simulink model "GVCU_HIL_simscape"  (R2026a)
settings: Solver=ode3  StartTime=0  StopTime=10  FixedStep=0.001
model workspace (MAT data in the model file):
  CANoelibParameters : object (value not decoded)
values from neighbouring files (symbols this model uses):
  acc_pedal_data = pedal_data.accelerator_pedal_position_t0    [Init_Simscape_main.m]
  acc_pedal_time = pedal_data.t0    [Init_Simscape_main.m]
  brk_pedal_data = brake_pedal_data.shared_brakes_drvrBrkPedlPerc_t0    [Init_Simscape_main.m]
  brk_pedal_time = brake_pedal_data.t0    [Init_Simscape_main.m]
  cycle_len = zeros(1, num_cycles)    [Init_Simscape_main.m]
  cycle_speed_matrix = zeros(max_cycle_len, num_cycles)    [Init_Simscape_main.m]
  cycle_time_matrix = zeros(max_cycle_len, num_cycles)    [Init_Simscape_main.m]
  veh_speed_data = speed_data.shared_dynamicsVso_vehVelLgt_t0    [Init_Simscape_main.m]
  veh_speed_time = speed_data.t0    [Init_Simscape_main.m]
undefined symbols (not defined in the file or in its folder): Active, aero, AuxActive, bat, brake, config, environment, FL, FL_prs_voltage, FR, FR_prs_voltage, front, pos, powertrain, rear, RL, RL_prs_voltage, RR, RR_prs_voltage, tir, veh, VGetRawValueFlag, Voltage, VT2816_1_Ch1, VT2816_1_Ch2, VT2816_1_Ch3, VT2816_1_Ch4, VT2816_3_Ch13, VT2816_3_Ch14, VT7101_1_Out2, VTS, X, Y, Z
libraries: sm_lib x358, fl_lib x272, nesl_utility x193, canoelib x127, sdl_lib x36, autolibsharedcoupling x21, autolibcoupling x9, slpidlib x7, simulink x3, autolibshareddiff x3, autolibshared x3, autolibutils x1
(part 10 of 17)

== system GVCU_HIL_simscape/GVCU - HiL/Commented messages/Message Output9 ==
  In1 : Inport
  Bus Selector : BusSelector  OutputSignals=charge_current,charge_port_status,charge_voltage,charging_mode,e2e_alive_counter_disabled,e2e_checksum_disabled,evcc_status,inlet_motor_status,obc_fan_req,obc_pump_req,obc_status
  S-Function_1 : S-Function  FunctionName=sigout  Parameters=dbName;nodeName;msgName;11;'charge_current';'charge_port_status';'charge_voltage';'charging_mode';'e2e_alive_counter_disabled';'e2e_checksum_disabled';'evcc_status';'inlet_motor_status';'obc_fan_req';'obc_pump_req';'obc_status';VGetRawValueFlag(rawValue);'inherited'  SFunctionDeploymentMode=off  EnableBusSupport=off
      settings: AttributesFormatString=charge_current\ncharge_port_status\ncharge_voltage\ncharging_mode\ne2e_alive_counter_disabled\ne2e_checksum_disabled\nevcc_status\ninlet_motor_status\nobc_fan_req\nobc_pump_req\nobc_status\n
  wires:
  In1/1 -> Bus Selector/1
  Bus Selector/1 -> S-Function_1/1  "<charge_current>"
  Bus Selector/2 -> S-Function_1/2  "<charge_port_status>"
  Bus Selector/3 -> S-Function_1/3  "<charge_voltage>"
  Bus Selector/4 -> S-Function_1/4  "<charging_mode>"
  Bus Selector/5 -> S-Function_1/5  "<e2e_alive_counter_disabled>"
  Bus Selector/6 -> S-Function_1/6  "<e2e_checksum_disabled>"
  Bus Selector/7 -> S-Function_1/7  "<evcc_status>"
  Bus Selector/8 -> S-Function_1/8  "<inlet_motor_status>"
  Bus Selector/9 -> S-Function_1/9  "<obc_fan_req>"
  Bus Selector/10 -> S-Function_1/10  "<obc_pump_req>"
  Bus Selector/11 -> S-Function_1/11  "<obc_status>"

== system GVCU_HIL_simscape/Powertrain (EV)/AWD_Powertrain1/Central axle ==
  Rear_axle_speed : Inport
  Tosional_rear_c : Inport  Port=2
  Central_Clutch : autolibcoupling/Disc Clutch  port_config=Simulink  Reff=.091/2  Ndisk=9  Aeff=0.006283185  Peng=320000  Jin=.1  Jout=.1  muk=.088  mus=.089  bin=.001  bout=.001  win_o=pos.xdot_0/veh.TyreLoadedRadius_F*veh.BevelGear_F  wout_o=pos.xdot_0/veh.TyreLoadedRadius_F*veh.BevelGear_F  tauC=.01  InitiallyLocked=off  maxAbsSpd=3000  blkID=1
  FR1 : autolibsharedcoupling/Torsional Compliance  port_config=Simulink  extInfo=off  k=5e4  b=4e2  theta_o=0  domega_o=0  omega_c=3000  blkID=0  aMode=1
  FR2 : autolibsharedcoupling/Torsional Compliance  port_config=Simulink  extInfo=off  k=5e4  b=4e2  theta_o=0  domega_o=0  omega_c=3000  blkID=0  aMode=1
  Gain1 : Gain  Gain=1/0.93
  Terminator : Terminator
  drop gear + omega_to_rpm_central : Gain  Gain=0.92 *30/pi
  Prop_shaft_trq : Outport
  Central_axle_trq : Outport  Port=2
  tag scope: third_shaft_spd=global
  wires:
  Central_Clutch/1 -> Terminator/1
  [Center_prs] -> Central_Clutch/1
  FR2/2 -> Central_Clutch/2
  Gain1/1 -> Prop_shaft_trq/1
  FR1/2 -> Gain1/1
  Tosional_rear_c/1 -> drop gear + omega_to_rpm_central/1, FR1/2
  FR2/1 -> Central_axle_trq/1
  FR1/1 -> Central_Clutch/3
  Central_Clutch/3 -> FR1/1
  Central_Clutch/2 -> FR2/2  "FrontSpd"
  Rear_axle_speed/1 -> FR2/1
  drop gear + omega_to_rpm_central/1 -> [third_shaft_spd]  "Front_axle_freq"

== system GVCU_HIL_simscape/Powertrain (EV)/AWD_Powertrain1/Front Axle ==
  AxlSpd : Inport
  Veh : Inport  Port=2
  Bus Selector : BusSelector  OutputSignals=Wheels.Omega
  Demux : Demux
  FL : autolibsharedcoupling/Torsional Compliance  port_config=Simulink  extInfo=off  k=5e4  b=4e2  theta_o=0  domega_o=0  omega_c=3000  blkID=0  aMode=1
  FL_Clutch : autolibcoupling/Disc Clutch  port_config=Simulink  Reff=.091/2  Ndisk=9  Aeff=0.006283185  Peng=320000  Jin=.1  Jout=.1  muk=.088  mus=.089  bin=.001  bout=.001  win_o=pos.xdot_0/veh.TyreLoadedRadius_F  wout_o=pos.xdot_0/veh.TyreLoadedRadius_F  tauC=1  InitiallyLocked=off  maxAbsSpd=3000  blkID=1
  FR : autolibsharedcoupling/Torsional Compliance  port_config=Simulink  extInfo=off  k=5e4  b=4e2  theta_o=0  domega_o=0  omega_c=3000  blkID=0  aMode=1
  FR_Clutch : autolibcoupling/Disc Clutch  port_config=Simulink  Reff=.091/2  Ndisk=9  Aeff=0.006283185  Peng=320000  Jin=.1  Jout=.1  muk=.088  mus=.089  bin=.001  bout=.001  win_o=pos.xdot_0/veh.TyreLoadedRadius_F  wout_o=pos.xdot_0/veh.TyreLoadedRadius_F  tauC=.01  InitiallyLocked=off  maxAbsSpd=3000  blkID=1
  Gain : Gain  Gain=1/2.71
  Split Torsional Compliance : autolibsharedcoupling/Split Torsional Compliance  port_config=Simulink  cplrMode=Shaft split  extInfo=off  k1=5e4  b1=4e2  omega1_c=1000  theta1_o=0  domega1_o=0  k2=5e4  b2=4e2  omega2_c=1000  theta2_o=0  domega2_o=0  blkID=0  aMode=1
      settings: LibrarySourceBlock=autolibcoupling/Split Torsional Compliance
  Terminator{,1..3} (4 alike) : Terminator
  omega_to_freq_FL : Gain  Gain=98/(2*pi)
  omega_to_freq_FR : Gain  Gain=98/(2*pi)
  Split torsional Compliance Trq : Outport
  Trq_FL : Outport  Port=2
  Trq_FR : Outport  Port=3
  tag scope: Axl_front_Spd=global, FL_G_Spd=global, FL_R_Spd=global, FL_sen=global, FR_G_Spd=global, FR_R_Spd=global, FR_sen=global, Split_tors_FL=global, Split_tors_FR=global
  wires:
  Split Torsional Compliance/1 -> Split torsional Compliance Trq/1
  FR/2 -> Trq_FR/1
  FL/2 -> Trq_FL/1
  FR/1 -> FR_Clutch/3
  FL/1 -> FL_Clutch/3
  FL_Clutch/1 -> Terminator3/1
  FR_Clutch/1 -> Terminator2/1
  FR_Clutch/2 -> Split Torsional Compliance/3
  FL_Clutch/2 -> Split Torsional Compliance/2
  Demux/2 -> [FR_G_Spd], FR/2
  FR_Clutch/3 -> omega_to_freq_FR/1, [FR_R_Spd], FR/1
  Demux/4 -> Terminator1/1
  Demux/3 -> Terminator/1
  Bus Selector/1 -> Demux/1  "<Omega>"
  Veh/1 -> Bus Selector/1
  FL_Clutch/3 -> omega_to_freq_FL/1, [FL_R_Spd], FL/1
  [FR_prs] -> FR_Clutch/1
  [FL_prs] -> FL_Clutch/1
  Split Torsional Compliance/2 -> [Split_tors_FL], FL_Clutch/2  "Front_left_clutch"
  AxlSpd/1 -> Gain/1
  Split Torsional Compliance/3 -> [Split_tors_FR], FR_Clutch/2  "Front_right_clutch"
  omega_to_freq_FL/1 -> [FL_sen]  "FL_freq"
  omega_to_freq_FR/1 -> [FR_sen]  "FR_freq"
  Demux/1 -> [FL_G_Spd], FL/2
  Gain/1 -> [Axl_front_Spd], Split Torsional Compliance/1  "Front axle"

== system GVCU_HIL_simscape/Powertrain (EV)/AWD_Powertrain1/Rear Axle ==
  Prop_shaft_trq : Inport
  Veh : Inport  Port=2
  Bus Selector : BusSelector  OutputSignals=Wheels.Omega
  Demux : Demux
  Gain{,1..3} (4 alike) : Gain  Gain=37/(2*pi)
  RL : autolibsharedcoupling/Torsional Compliance  port_config=Simulink  extInfo=off  k=8e4  b=4e2  theta_o=0  domega_o=0  omega_c=3000  blkID=0  aMode=1
  RL_Clutch : autolibcoupling/Disc Clutch  port_config=Simulink  Reff=.091/2  Ndisk=9  Aeff=0.006283185  Peng=320000  Jin=.1  Jout=.1  muk=.088  mus=.089  bin=.001  bout=.001  win_o=pos.xdot_0/veh.TyreLoadedRadius_R*veh.RearSideGear  wout_o=pos.xdot_0/veh.TyreLoadedRadius_R*veh.RearSideGear  tauC=.01  InitiallyLocked=off  maxAbsSpd=3000  blkID=1
  RL_SideGearbox : autolibsharedcoupling/Gearbox  port_config=Simulink  input_config=Torque input - velocity output  DiffEffModelPopup=Constant  InterpMethod=Flat  dirSwitch=on  extTamb=off  N=veh.RearSideGear  J1=.01  J2=.01  b1=.001  b2=.001  theta1_o=0  w1_o=pos.xdot_0/veh.TyreLoadedRadius_R*veh.RearSideGear  eta=1  eta_tbl=reshape([0.64 0.76 0.8 0.81 0.83 0.84 0.84 0.56 0.73 0.78 0.8 0.83 0.84 0.84 0.54 0.71 0.77 0.8 0.82 0.84 0.84 0.53 0.71 0.77 0.8 0.83 0.84 0.84 0.51 0.71 0.77 0.8 0.83 0.84 0.85 0.52 0.7 0.77 0.8 0.83 0.84 0.85 0.51 0.71 0.76 0.79 0.83 0.84 0.85 0.5 0.69 0.76 0.79 0.82 0.84 0.85 0.45 0.68 0.75 0.78 0.82 0.84 0.85 0.43 0.67 0.74 0.78 0.81 0.83 0.84 0.38 0.63 0.71 0.75 0.8 0.82 0.83 0.81 0.86 0.88 0.89 0.89 0.89 0.9 0.77 0.85 0.87 0.88 0.89 0.9 0.9 0.72 0.82 0.86 0.87 0.88 0.89 0.9 0.68 0.8 0.84 0.86 0.88 0.89 0.89 0.67 0.8 0.84 0.86 0.88 0.89 0.9 0.67 0.8 0.84 0.86 0.88 0.89 0.9 0.65 0.8 0.84 0.86 0.88 0.89 0.9 0.64 0.79 0.83 0.86 0.88 0.89 0.9 0.63 0.78 0.83 0.86 0.88 0.89 0.9 0.59 0.76 0.82 0.85 0.87 0.89 0.9 0.53 0.73 0.8 0.83 0.86 0.88 0.89], 7, 11, 2)  Trq_bpts=[25, 50, 75, 100, 150, 200, 250]  omega_bpts=[52.4 78.5 105 131 157 183 209 262 314 419 524]  Temp_bpts=[290 358]  Tamb=297.15  blkID=0  aMode=1
  RL_clutch_c : autolibsharedcoupling/Torsional Compliance  port_config=Simulink  extInfo=off  k=4e4  b=1e2  theta_o=0  domega_o=0  omega_c=3000  blkID=0  aMode=1
  RR : autolibsharedcoupling/Torsional Compliance  port_config=Simulink  extInfo=off  k=8e4  b=4e2  theta_o=0  domega_o=0  omega_c=3000  blkID=0  aMode=1
  RR_Clutch : autolibcoupling/Disc Clutch  port_config=Simulink  Reff=.091/2  Ndisk=9  Aeff=0.006283185  Peng=320000  Jin=.1  Jout=.1  muk=.088  mus=.089  bin=.001  bout=.001  win_o=pos.xdot_0/veh.TyreLoadedRadius_R*veh.RearSideGear  wout_o=pos.xdot_0/veh.TyreLoadedRadius_R*veh.RearSideGear  tauC=.01  InitiallyLocked=off  maxAbsSpd=3000  blkID=1
  RR_SideGearbox : autolibsharedcoupling/Gearbox  port_config=Simulink  input_config=Torque input - velocity output  DiffEffModelPopup=Constant  InterpMethod=Flat  dirSwitch=on  extTamb=off  N=2.38  J1=.01  J2=.01  b1=.001  b2=.001  theta1_o=0  w1_o=pos.xdot_0/veh.TyreLoadedRadius_R*veh.RearSideGear  eta=1  eta_tbl=reshape([0.64 0.76 0.8 0.81 0.83 0.84 0.84 0.56 0.73 0.78 0.8 0.83 0.84 0.84 0.54 0.71 0.77 0.8 0.82 0.84 0.84 0.53 0.71 0.77 0.8 0.83 0.84 0.84 0.51 0.71 0.77 0.8 0.83 0.84 0.85 0.52 0.7 0.77 0.8 0.83 0.84 0.85 0.51 0.71 0.76 0.79 0.83 0.84 0.85 0.5 0.69 0.76 0.79 0.82 0.84 0.85 0.45 0.68 0.75 0.78 0.82 0.84 0.85 0.43 0.67 0.74 0.78 0.81 0.83 0.84 0.38 0.63 0.71 0.75 0.8 0.82 0.83 0.81 0.86 0.88 0.89 0.89 0.89 0.9 0.77 0.85 0.87 0.88 0.89 0.9 0.9 0.72 0.82 0.86 0.87 0.88 0.89 0.9 0.68 0.8 0.84 0.86 0.88 0.89 0.89 0.67 0.8 0.84 0.86 0.88 0.89 0.9 0.67 0.8 0.84 0.86 0.88 0.89 0.9 0.65 0.8 0.84 0.86 0.88 0.89 0.9 0.64 0.79 0.83 0.86 0.88 0.89 0.9 0.63 0.78 0.83 0.86 0.88 0.89 0.9 0.59 0.76 0.82 0.85 0.87 0.89 0.9 0.53 0.73 0.8 0.83 0.86 0.88 0.89], 7, 11, 2)  Trq_bpts=[25, 50, 75, 100, 150, 200, 250]  omega_bpts=[52.4 78.5 105 131 157 183 209 262 314 419 524]  Temp_bpts=[290 358]  Tamb=297.15  blkID=0  aMode=1
  RR_clutch_c : autolibsharedcoupling/Torsional Compliance  port_config=Simulink  extInfo=off  k=4e4  b=1e2  theta_o=0  domega_o=0  omega_c=3000  blkID=0  aMode=1
  Rear_left_split : autolibsharedcoupling/Torsional Compliance  port_config=Simulink  extInfo=off  k=4e4  b=1e2  theta_o=0  domega_o=0  omega_c=3000  blkID=0  aMode=1
  Rear_right_split : autolibsharedcoupling/Torsional Compliance  port_config=Simulink  extInfo=off  k=4e4  b=1e2  theta_o=0  domega_o=0  omega_c=3000  blkID=0  aMode=1
  Terminator{,1..6} (7 alike) : Terminator
  Transfer Case : autolibshareddiff/Transfer Case  DiffEffModelPopup=Constant  InterpMethod=Linear point-slope  extTamb=off  TrqSplitRatioMode=off  SpdLockMode=off  shaftSwitchMask=To the left of center-line  Ndiff=veh.BevelGear_R  Jd=.1  bd=1e-3  Jw1=.1  bw1=1e-3  Jw2=.1  bw2=1e-3  omegaw1o=pos.xdot_0/veh.TyreLoadedRadius_R*veh.RearSideGear  omegaw2o=pos.xdot_0/veh.TyreLoadedRadius_R*veh.RearSideGear  eta=1  eta_tbl=reshape([0.64 0.76 0.8 0.81 0.83 0.84 0.84 0.56 0.73 0.78 0.8 0.83 0.84 0.84 0.54 0.71 0.77 0.8 0.82 0.84 0.84 0.53 0.71 0.77 0.8 0.83 0.84 0.84 0.51 0.71 0.77 0.8 0.83 0.84 0.85 0.52 0.7 0.77 0.8 0.83 0.84 0.85 0.51 0.71 0.76 0.79 0.83 0.84 0.85 0.5 0.69 0.76 0.79 0.82 0.84 0.85 0.45 0.68 0.75 0.78 0.82 0.84 0.85 0.43 0.67 0.74 0.78 0.81 0.83 0.84 0.38 0.63 0.71 0.75 0.8 0.82 0.83 0.81 0.86 0.88 0.89 0.89 0.89 0.9 0.77 0.85 0.87 0.88 0.89 0.9 0.9 0.72 0.82 0.86 0.87 0.88 0.89 0.9 0.68 0.8 0.84 0.86 0.88 0.89 0.89 0.67 0.8 0.84 0.86 0.88 0.89 0.9 0.67 0.8 0.84 0.86 0.88 0.89 0.9 0.65 0.8 0.84 0.86 0.88 0.89 0.9 0.64 0.79 0.83 0.86 0.88 0.89 0.9 0.63 0.78 0.83 0.86 0.88 0.89 0.9 0.59 0.76 0.82 0.85 0.87 0.89 0.9 0.53 0.73 0.8 0.83 0.86 0.88 0.89], 7, 11, 2)  Trq_bpts=[25, 50, 75, 100, 150, 200, 250]  omega_bpts=[52.4 78.5 105 131 157 183 209 262 314 419 524]  Temp_bpts=[290 358]  Tamb=297.15  maxAbsSpd=5e3  aMode=1  TrqSplitRatio=0.5  SpdLock=1
      settings: LibrarySourceBlock=autolibdiff/Transfer Case
  Trq_RL : Outport
  Trq_RR : Outport  Port=2
  Tosional_rear_c : Outport  Port=3
  tag scope: RL_SenA=global, RL_senB=global, RR_SenA=global, RR_senB=global
  wires:
  Transfer Case/2 -> Tosional_rear_c/1  "DriveshaftSpd"
  Demux/4 -> RR/2
  Demux/3 -> RL/2
  Demux/1 -> Terminator6/1
  Bus Selector/1 -> Demux/1  "<Omega>"
  Demux/2 -> Terminator5/1
  Veh/1 -> Bus Selector/1
  RR_SideGearbox/1 -> Terminator4/1
  RR/1 -> RR_SideGearbox/2
  RL/1 -> RL_SideGearbox/2
  RR/2 -> Trq_RR/1  "SG_RR"
  RL/2 -> Trq_RL/1  "SG_RL"
  RR_SideGearbox/3 -> RR/1  "w_RR"
  RR_clutch_c/1 -> RR_Clutch/3
  RR_SideGearbox/2 -> RR_clutch_c/2
  RR_clutch_c/2 -> RR_SideGearbox/1  "VT_RR"
  RR_Clutch/3 -> Gain3/1, Gain2/1, RR_clutch_c/1
  RR_Clutch/2 -> Rear_right_split/2
  RL_Clutch/2 -> Rear_left_split/2
  RL_SideGearbox/1 -> Terminator3/1
  RL_SideGearbox/2 -> RL_clutch_c/2
  RL_SideGearbox/3 -> RL/1  "w_RL"
  RL_clutch_c/2 -> RL_SideGearbox/1  "VT_RL"
  RL_clutch_c/1 -> RL_Clutch/3
  RL_Clutch/3 -> Gain1/1, Gain/1, RL_clutch_c/1
  RR_Clutch/1 -> Terminator2/1
  RL_Clutch/1 -> Terminator1/1
  [RR_prs] -> RR_Clutch/1
  [RL_prs] -> RL_Clutch/1
  Rear_right_split/2 -> RR_Clutch/2
  Rear_right_split/1 -> Transfer Case/3
  Rear_left_split/1 -> Transfer Case/2
  Rear_left_split/2 -> RL_Clutch/2
  Transfer Case/4 -> Rear_right_split/1  "Axl1Spd"
  Transfer Case/3 -> Rear_left_split/1
  Transfer Case/1 -> Terminator/1
  Prop_shaft_trq/1 -> Transfer Case/1
  Gain/1 -> [RL_SenA]  "RL_freq_A"
  Gain1/1 -> [RL_senB]  "RL_freq_B"
  Gain3/1 -> [RR_senB]  "RR_freq_B"
  Gain2/1 -> [RR_SenA]  "RR_freq_A"

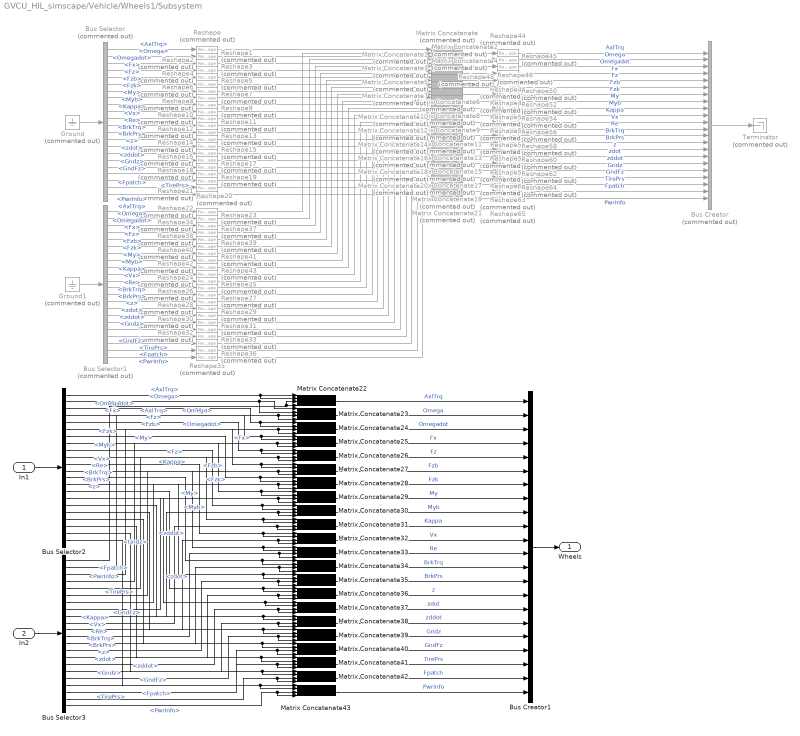
== system GVCU_HIL_simscape/Vehicle/Wheels1/Subsystem ==
  In1 : Inport
  In2 : Inport  Port=2
  Bus Creator : BusCreator  Commented=on  Inputs=22
  Bus Creator1 : BusCreator  Inputs=22
  Bus Selector : BusSelector  Commented=on  OutputSignals=AxlTrq,Omega,Omegadot,Fx,Fz,Fzb,Fzk,My,Myb,Kappa,Vx,Re,BrkTrq,BrkPrs,z,zdot,zddot,Gndz,GndFz,TirePrs,Fpatch,PwrInfo
  Bus Selector1 : BusSelector  Commented=on  OutputSignals=AxlTrq,Omega,Omegadot,Fx,Fz,Fzb,Fzk,My,Myb,Kappa,Vx,Re,BrkTrq,BrkPrs,z,zdot,zddot,Gndz,GndFz,TirePrs,Fpatch,PwrInfo
  Bus Selector2 : BusSelector  OutputSignals=AxlTrq,Omega,Omegadot,Fx,Fz,Fzb,Fzk,My,Myb,Kappa,Vx,Re,BrkTrq,BrkPrs,z,zdot,zddot,Gndz,GndFz,TirePrs,Fpatch,PwrInfo
  Bus Selector3 : BusSelector  OutputSignals=AxlTrq,Omega,Omegadot,Fx,Fz,Fzb,Fzk,My,Myb,Kappa,Vx,Re,BrkTrq,BrkPrs,z,zdot,zddot,Gndz,GndFz,TirePrs,Fpatch,PwrInfo
  Ground : Ground  Commented=on
  Ground1 : Ground  Commented=on
  Matrix Concatenate : Concatenate  Commented=on
  Matrix Concatenate{1..21} (21 alike) : Concatenate  Commented=on  ConcatenateDimension=2
  Matrix Concatenate{22..43} (22 alike) : Concatenate  NumInputs=4
  Reshape{,1..43} (44 alike) : Reshape  Commented=on  OutputDimensionality=Row vector (2-D)
  Reshape{44..65} (22 alike) : Reshape  Commented=on
  Terminator : Terminator  Commented=on
  Wheels : Outport
  wires:
  Bus Selector/1 -> Reshape/1  "<AxlTrq>"
  In2/1 -> Bus Selector3/1
  In1/1 -> Bus Selector2/1
  Bus Selector3/22 -> Matrix Concatenate43/3, Matrix Concatenate43/4  "<PwrInfo>"
  Bus Selector3/21 -> Matrix Concatenate42/3, Matrix Concatenate42/4  "<Fpatch>"
  Bus Selector3/20 -> Matrix Concatenate41/3, Matrix Concatenate41/4  "<TirePrs>"
  Bus Selector3/19 -> Matrix Concatenate40/3, Matrix Concatenate40/4  "<GndFz>"
  Bus Selector3/18 -> Matrix Concatenate39/3, Matrix Concatenate39/4  "<Gndz>"
  Bus Selector3/17 -> Matrix Concatenate38/3, Matrix Concatenate38/4  "<zddot>"
  Bus Selector3/16 -> Matrix Concatenate37/3, Matrix Concatenate37/4  "<zdot>"
  Bus Selector3/15 -> Matrix Concatenate36/3, Matrix Concatenate36/4  "<z>"
  Bus Selector3/14 -> Matrix Concatenate35/3, Matrix Concatenate35/4  "<BrkPrs>"
  Bus Selector3/13 -> Matrix Concatenate34/3, Matrix Concatenate34/4  "<BrkTrq>"
  Bus Selector3/12 -> Matrix Concatenate33/3, Matrix Concatenate33/4  "<Re>"
  Bus Selector3/11 -> Matrix Concatenate32/3, Matrix Concatenate32/4  "<Vx>"
  Bus Selector3/10 -> Matrix Concatenate31/3, Matrix Concatenate31/4  "<Kappa>"
  Bus Selector3/9 -> Matrix Concatenate30/3, Matrix Concatenate30/4  "<Myb>"
  Bus Selector3/8 -> Matrix Concatenate29/3, Matrix Concatenate29/4  "<My>"
  Bus Selector3/7 -> Matrix Concatenate28/3, Matrix Concatenate28/4  "<Fzk>"
  Bus Selector3/6 -> Matrix Concatenate27/3, Matrix Concatenate27/4  "<Fzb>"
  Bus Selector3/5 -> Matrix Concatenate26/3, Matrix Concatenate26/4  "<Fz>"
  Bus Selector3/4 -> Matrix Concatenate25/3, Matrix Concatenate25/4  "<Fx>"
  Bus Selector3/3 -> Matrix Concatenate24/3, Matrix Concatenate24/4  "<Omegadot>"
  Bus Selector3/2 -> Matrix Concatenate23/3, Matrix Concatenate23/4  "<Omega>"
  Bus Selector3/1 -> Matrix Concatenate22/3, Matrix Concatenate22/4  "<AxlTrq>"
  Matrix Concatenate23/1 -> Bus Creator1/2  "Omega"
  Matrix Concatenate29/1 -> Bus Creator1/8  "My"
  Matrix Concatenate36/1 -> Bus Creator1/15  "z"
  Matrix Concatenate27/1 -> Bus Creator1/6  "Fzb"
  Matrix Concatenate25/1 -> Bus Creator1/4  "Fx"
  Matrix Concatenate33/1 -> Bus Creator1/12  "Re"
  Matrix Concatenate28/1 -> Bus Creator1/7  "Fzk"
  Matrix Concatenate30/1 -> Bus Creator1/9  "Myb"
  Matrix Concatenate31/1 -> Bus Creator1/10  "Kappa"
  Matrix Concatenate43/1 -> Bus Creator1/22  "Pwrinfo"
  Matrix Concatenate22/1 -> Bus Creator1/1  "AxlTrq"
  Matrix Concatenate38/1 -> Bus Creator1/17  "zddot"
  Matrix Concatenate37/1 -> Bus Creator1/16  "zdot"
  Matrix Concatenate41/1 -> Bus Creator1/20  "TirePrs"
  Matrix Concatenate39/1 -> Bus Creator1/18  "Gndz"
  Matrix Concatenate24/1 -> Bus Creator1/3  "Omegadot"
  Matrix Concatenate26/1 -> Bus Creator1/5  "Fz"
  Matrix Concatenate35/1 -> Bus Creator1/14  "BrkPrs"
  Matrix Concatenate42/1 -> Bus Creator1/21  "Fpatch"
  Matrix Concatenate40/1 -> Bus Creator1/19  "GndFz"
  Matrix Concatenate34/1 -> Bus Creator1/13  "BrkTrq"
  Matrix Concatenate32/1 -> Bus Creator1/11  "Vx"
  Bus Creator1/1 -> Wheels/1
  Bus Selector2/22 -> Matrix Concatenate43/2, Matrix Concatenate43/1  "<PwrInfo>"
  Bus Selector2/21 -> Matrix Concatenate42/1, Matrix Concatenate42/2  "<Fpatch>"
  Bus Selector2/20 -> Matrix Concatenate41/1, Matrix Concatenate41/2  "<TirePrs>"
  Bus Selector2/19 -> Matrix Concatenate40/1, Matrix Concatenate40/2  "<GndFz>"
  Bus Selector2/18 -> Matrix Concatenate39/1, Matrix Concatenate39/2  "<Gndz>"
  Bus Selector2/17 -> Matrix Concatenate38/1, Matrix Concatenate38/2  "<zddot>"
  Bus Selector2/16 -> Matrix Concatenate37/1, Matrix Concatenate37/2  "<zdot>"
  Bus Selector2/15 -> Matrix Concatenate36/1, Matrix Concatenate36/2  "<z>"
  Bus Selector2/14 -> Matrix Concatenate35/1, Matrix Concatenate35/2  "<BrkPrs>"
  Bus Selector2/13 -> Matrix Concatenate34/2, Matrix Concatenate34/1  "<BrkTrq>"
  Bus Selector2/12 -> Matrix Concatenate33/1, Matrix Concatenate33/2  "<Re>"
  Bus Selector2/11 -> Matrix Concatenate32/2, Matrix Concatenate32/1  "<Vx>"
  Bus Selector2/10 -> Matrix Concatenate31/1, Matrix Concatenate31/2  "<Kappa>"
  Bus Selector2/9 -> Matrix Concatenate30/1, Matrix Concatenate30/2  "<Myb>"
  Bus Selector2/8 -> Matrix Concatenate29/1, Matrix Concatenate29/2  "<My>"
  Bus Selector2/7 -> Matrix Concatenate28/1, Matrix Concatenate28/2  "<Fzk>"
  Bus Selector2/6 -> Matrix Concatenate27/1, Matrix Concatenate27/2  "<Fzb>"
  Bus Selector2/5 -> Matrix Concatenate26/1, Matrix Concatenate26/2  "<Fz>"
  Bus Selector2/4 -> Matrix Concatenate25/1, Matrix Concatenate25/2  "<Fx>"
  Bus Selector2/3 -> Matrix Concatenate24/2, Matrix Concatenate24/1  "<Omegadot>"
  Bus Selector2/2 -> Matrix Concatenate23/2, Matrix Concatenate23/1  "<Omega>"
  Bus Selector2/1 -> Matrix Concatenate22/1, Matrix Concatenate22/2  "<AxlTrq>"
  Bus Creator/1 -> Terminator/1
  Reshape56/1 -> Bus Creator/13  "BrkTrq"
  Reshape54/1 -> Bus Creator/11  "Vx"
  Reshape55/1 -> Bus Creator/12  "Re"
  Reshape57/1 -> Bus Creator/14  "BrkPrs"
  Reshape58/1 -> Bus Creator/15  "z"
  Reshape59/1 -> Bus Creator/16  "zdot"
  Reshape60/1 -> Bus Creator/17  "zddot"
  Reshape61/1 -> Bus Creator/18  "Gndz"
  Reshape62/1 -> Bus Creator/19  "GndFz"
  Reshape63/1 -> Bus Creator/20  "TirePrs"
  Reshape64/1 -> Bus Creator/21  "Fpatch"
  Reshape65/1 -> Bus Creator/22  "Pwrinfo"
  Reshape53/1 -> Bus Creator/10  "Kappa"
  Reshape52/1 -> Bus Creator/9  "Myb"
  Reshape51/1 -> Bus Creator/8  "My"
  Reshape50/1 -> Bus Creator/7  "Fzk"
  Reshape49/1 -> Bus Creator/6  "Fzb"
  Reshape48/1 -> Bus Creator/5  "Fz"
  Reshape47/1 -> Bus Creator/4  "Fx"
  Reshape46/1 -> Bus Creator/3  "Omegadot"
  Reshape45/1 -> Bus Creator/2  "Omega"
  Reshape44/1 -> Bus Creator/1  "AxlTrq"
  Matrix Concatenate21/1 -> Reshape65/1
  Matrix Concatenate20/1 -> Reshape64/1
  Matrix Concatenate19/1 -> Reshape63/1
  Matrix Concatenate18/1 -> Reshape62/1
  Matrix Concatenate17/1 -> Reshape61/1
  Matrix Concatenate16/1 -> Reshape60/1
  Matrix Concatenate15/1 -> Reshape59/1
  Matrix Concatenate14/1 -> Reshape58/1
  Matrix Concatenate13/1 -> Reshape57/1
  Matrix Concatenate12/1 -> Reshape56/1
  Matrix Concatenate11/1 -> Reshape55/1
  Matrix Concatenate10/1 -> Reshape54/1
  Matrix Concatenate9/1 -> Reshape53/1
  Matrix Concatenate8/1 -> Reshape52/1
  Matrix Concatenate7/1 -> Reshape51/1
  Matrix Concatenate6/1 -> Reshape50/1
  Matrix Concatenate5/1 -> Reshape49/1
  Matrix Concatenate4/1 -> Reshape48/1
  Matrix Concatenate3/1 -> Reshape47/1
  Matrix Concatenate2/1 -> Reshape46/1
  Matrix Concatenate1/1 -> Reshape45/1
  Matrix Concatenate/1 -> Reshape44/1
  Reshape25/1 -> Matrix Concatenate11/2
  Reshape26/1 -> Matrix Concatenate12/2
  Reshape27/1 -> Matrix Concatenate13/2
  Reshape28/1 -> Matrix Concatenate14/2
  Reshape29/1 -> Matrix Concatenate15/2
  Reshape30/1 -> Matrix Concatenate16/2
  Reshape31/1 -> Matrix Concatenate17/2
  Reshape32/1 -> Matrix Concatenate18/2
  Reshape33/1 -> Matrix Concatenate19/2
  Reshape35/1 -> Matrix Concatenate20/2
  Reshape36/1 -> Matrix Concatenate21/2
  Reshape24/1 -> Matrix Concatenate10/2
  Reshape43/1 -> Matrix Concatenate9/2
  Reshape42/1 -> Matrix Concatenate8/2
  Reshape41/1 -> Matrix Concatenate7/2
  Reshape40/1 -> Matrix Concatenate6/2
  Reshape39/1 -> Matrix Concatenate5/2
  Reshape21/1 -> Matrix Concatenate21/1
  Reshape20/1 -> Matrix Concatenate20/1
  Reshape19/1 -> Matrix Concatenate19/1
  Reshape18/1 -> Matrix Concatenate18/1
  Reshape17/1 -> Matrix Concatenate17/1
  Reshape16/1 -> Matrix Concatenate16/1
  Reshape15/1 -> Matrix Concatenate15/1
  Reshape14/1 -> Matrix Concatenate14/1
  Reshape13/1 -> Matrix Concatenate13/1
  Reshape12/1 -> Matrix Concatenate12/1
  Reshape11/1 -> Matrix Concatenate11/1
  Reshape10/1 -> Matrix Concatenate10/1
  Reshape9/1 -> Matrix Concatenate9/1
  Reshape8/1 -> Matrix Concatenate8/1
  Reshape7/1 -> Matrix Concatenate7/1
  Reshape6/1 -> Matrix Concatenate6/1
  Reshape5/1 -> Matrix Concatenate5/1
  Reshape38/1 -> Matrix Concatenate4/2
  Reshape37/1 -> Matrix Concatenate3/2
  Reshape4/1 -> Matrix Concatenate4/1
  Reshape3/1 -> Matrix Concatenate3/1
  Reshape34/1 -> Matrix Concatenate2/2
  Reshape2/1 -> Matrix Concatenate2/1
  Reshape23/1 -> Matrix Concatenate1/2
  Reshape1/1 -> Matrix Concatenate1/1
  Reshape22/1 -> Matrix Concatenate/2
  Reshape/1 -> Matrix Concatenate/1
  Bus Selector1/19 -> Reshape32/1  "<GndFz>"
  Bus Selector1/13 -> Reshape26/1  "<BrkTrq>"
  Bus Selector1/15 -> Reshape28/1  "<z>"
  Bus Selector1/5 -> Reshape38/1  "<Fz>"
  Ground1/1 -> Bus Selector1/1
  Bus Selector1/14 -> Reshape27/1  "<BrkPrs>"
  Bus Selector1/1 -> Reshape22/1  "<AxlTrq>"
  Bus Selector1/10 -> Reshape43/1  "<Kappa>"
  Bus Selector1/6 -> Reshape39/1  "<Fzb>"
  Bus Selector1/11 -> Reshape24/1  "<Vx>"
  Bus Selector1/18 -> Reshape31/1  "<Gndz>"
  Bus Selector1/8 -> Reshape41/1  "<My>"
  Bus Selector1/22 -> Reshape36/1  "<PwrInfo>"
  Bus Selector1/21 -> Reshape35/1  "<Fpatch>"
  Bus Selector1/17 -> Reshape30/1  "<zddot>"
  Bus Selector1/2 -> Reshape23/1  "<Omega>"
  Bus Selector1/12 -> Reshape25/1  "<Re>"
  Bus Selector1/20 -> Reshape33/1  "<TirePrs>"
  Bus Selector1/9 -> Reshape42/1  "<Myb>"
  Bus Selector1/16 -> Reshape29/1  "<zdot>"
  Bus Selector1/7 -> Reshape40/1  "<Fzk>"
  Bus Selector1/3 -> Reshape34/1  "<Omegadot>"
  Bus Selector1/4 -> Reshape37/1  "<Fx>"
  Bus Selector/22 -> Reshape21/1  "<PwrInfo>"
  Bus Selector/21 -> Reshape20/1  "<Fpatch>"
  Bus Selector/20 -> Reshape19/1  "<TirePrs>"
  Bus Selector/19 -> Reshape18/1  "<GndFz>"
  Bus Selector/18 -> Reshape17/1  "<Gndz>"
  Bus Selector/17 -> Reshape16/1  "<zddot>"
  Bus Selector/16 -> Reshape15/1  "<zdot>"
  Bus Selector/15 -> Reshape14/1  "<z>"
  Bus Selector/14 -> Reshape13/1  "<BrkPrs>"
  Bus Selector/13 -> Reshape12/1  "<BrkTrq>"
  Bus Selector/12 -> Reshape11/1  "<Re>"
  Bus Selector/11 -> Reshape10/1  "<Vx>"
  Bus Selector/10 -> Reshape9/1  "<Kappa>"
  Bus Selector/9 -> Reshape8/1  "<Myb>"
  Bus Selector/8 -> Reshape7/1  "<My>"
  Bus Selector/7 -> Reshape6/1  "<Fzk>"
  Bus Selector/6 -> Reshape5/1  "<Fzb>"
  Bus Selector/5 -> Reshape4/1  "<Fz>"
  Bus Selector/4 -> Reshape3/1  "<Fx>"
  Bus Selector/3 -> Reshape2/1  "<Omegadot>"
  Bus Selector/2 -> Reshape1/1  "<Omega>"
  Ground/1 -> Bus Selector/1

== system GVCU_HIL_simscape/Vehicle/Wheels1/whel to axel transform3 ==
  Input (1x4) : Inport
  Selector4 : Selector  InputPortWidth=4  IndexOptions=Index vector (dialog)  Indices=[1]  OutputSizes=1
  Selector5 : Selector  InputPortWidth=4  IndexOptions=Index vector (dialog)  Indices=[2]  OutputSizes=1
  Selector6 : Selector  InputPortWidth=4  IndexOptions=Index vector (dialog)  Indices=[3]  OutputSizes=1
  Selector7 : Selector  InputPortWidth=4  IndexOptions=Index vector (dialog)  Indices=[4]  OutputSizes=1
  "Front L " : Outport
  Front R : Outport  Port=2
  "Rear L " : Outport  Port=3
  Rear R : Outport  Port=4
  wires:
  Selector7/1 -> Rear R/1
  Selector6/1 -> "Rear L "/1
  Selector5/1 -> Front R/1
  Selector4/1 -> "Front L "/1
  Input (1x4)/1 -> Selector4/1, Selector5/1, Selector7/1, Selector6/1

== system GVCU_HIL_simscape/vehicle/multibody/ARB ==
  Bus Creator : BusCreator  Inputs=2
  From : From
  Goto4 : Goto
  PS Divide{,1..3} (4 alike) : fl_lib/Physical Signals/Functions/PS Divide
  PS Gain1 : fl_lib/Physical Signals/Functions/PS Gain  gain=-1
  PS Product : fl_lib/Physical Signals/Functions/PS Product
  PS Subtract : fl_lib/Physical Signals/Functions/PS Subtract
  PS-Simulink Converter2 : nesl_utility/PS-Simulink Converter  PhysicalDomain=network_engine_domain  SubClassName=ps_output  LeftPortType=input  RightPortType=output  PseudoPeriodic=off  Frequencies=[]  VectorFormat=inherit  Unit=inherit  AffineConversion=off
  PS-Simulink Converter7 : nesl_utility/PS-Simulink Converter  PhysicalDomain=network_engine_domain  SubClassName=ps_output  LeftPortType=input  RightPortType=output  PseudoPeriodic=off  Frequencies=[]  VectorFormat=inherit  Unit=inherit  AffineConversion=off
  motion ratio left : fl_lib/Physical Signals/Lookup Tables/PS Lookup Table (1D)  x=front.z_bp m  f=front.ARB.mr_bp  interp_method=simscape.enum.interpolation.linear  extrap_method=simscape.enum.extrapolation.nearest
  motion ratio right : fl_lib/Physical Signals/Lookup Tables/PS Lookup Table (1D)  x=front.z_bp m  f=front.ARB.mr_bp  interp_method=simscape.enum.interpolation.linear  extrap_method=simscape.enum.extrapolation.nearest
  stiffness : fl_lib/Physical Signals/Sources/PS Constant  constant=front.ARB.k N/m
  pz_left : PMIOPort  Side=Left
  left : PMIOPort  Port=2  Side=Left
  pz_right : PMIOPort  Port=3  Side=Right
  right : PMIOPort  Port=4  Side=Right
  meas : Outport
  wires:
  [B] -> Bus Creator/2  "aARBTwist"
  Bus Creator/1 -> meas/1
  From/1 -> Bus Creator/1  "MARBTwist"
  PS-Simulink Converter7/1 -> Goto4/1
  PS-Simulink Converter2/1 -> [B]
  connections:
  motion ratio right/LConn1 -- pz_right/RConn1 -- PS Divide/LConn1
  motion ratio left/LConn1 -- pz_left/RConn1 -- PS Divide1/LConn1
  motion ratio right/RConn1 -- PS Divide2/LConn2 -- PS Divide/LConn2
  motion ratio left/RConn1 -- PS Divide3/LConn2 -- PS Divide1/LConn2
  PS Subtract/LConn1 -- PS Divide1/RConn1
  PS Divide/RConn1 -- PS Subtract/LConn2
  PS Product/LConn1 -- PS-Simulink Converter7/LConn1 -- PS Subtract/RConn1
  stiffness/RConn1 -- PS Product/LConn2
  PS Divide2/LConn1 -- PS Divide3/LConn1 -- PS-Simulink Converter2/LConn1 -- PS Product/RConn1
  PS Divide3/RConn1 -- PS Gain1/LConn1
  right/RConn1 -- PS Divide2/RConn1
  PS Gain1/RConn1 -- left/RConn1

== system GVCU_HIL_simscape/vehicle/multibody/ARB1 ==
  Bus Creator : BusCreator  Inputs=2
  From : From
  Goto4 : Goto
  PS Divide{,1..3} (4 alike) : fl_lib/Physical Signals/Functions/PS Divide
  PS Gain1 : fl_lib/Physical Signals/Functions/PS Gain  gain=-1
  PS Product : fl_lib/Physical Signals/Functions/PS Product
  PS Subtract : fl_lib/Physical Signals/Functions/PS Subtract
  PS-Simulink Converter2 : nesl_utility/PS-Simulink Converter  PhysicalDomain=network_engine_domain  SubClassName=ps_output  LeftPortType=input  RightPortType=output  PseudoPeriodic=off  Frequencies=[]  VectorFormat=inherit  Unit=inherit  AffineConversion=off
  PS-Simulink Converter7 : nesl_utility/PS-Simulink Converter  PhysicalDomain=network_engine_domain  SubClassName=ps_output  LeftPortType=input  RightPortType=output  PseudoPeriodic=off  Frequencies=[]  VectorFormat=inherit  Unit=inherit  AffineConversion=off
  motion ratio left : fl_lib/Physical Signals/Lookup Tables/PS Lookup Table (1D)  x=rear.z_bp m  f=rear.ARB.mr_bp  interp_method=simscape.enum.interpolation.linear  extrap_method=simscape.enum.extrapolation.nearest
  motion ratio right : fl_lib/Physical Signals/Lookup Tables/PS Lookup Table (1D)  x=rear.z_bp m  f=rear.ARB.mr_bp  interp_method=simscape.enum.interpolation.linear  extrap_method=simscape.enum.extrapolation.nearest
  stiffness : fl_lib/Physical Signals/Sources/PS Constant  constant=rear.ARB.k N/m
  left : PMIOPort  Side=Left
  pz_left : PMIOPort  Port=2  Side=Left
  right : PMIOPort  Port=3  Side=Right
  pz_right : PMIOPort  Port=4  Side=Right
  meas : Outport
  wires:
  [B] -> Bus Creator/2  "aARBTwist"
  Bus Creator/1 -> meas/1
  From/1 -> Bus Creator/1  "MARBTwist"
  PS-Simulink Converter7/1 -> Goto4/1
  PS-Simulink Converter2/1 -> [B]
  connections:
  PS Divide2/LConn1 -- PS Divide3/LConn1 -- PS-Simulink Converter2/LConn1 -- PS Product/RConn1
  motion ratio left/LConn1 -- pz_left/RConn1 -- PS Divide1/LConn1
  motion ratio right/LConn1 -- pz_right/RConn1 -- PS Divide/LConn1
  PS Divide1/LConn2 -- motion ratio left/RConn1 -- PS Divide3/LConn2
  motion ratio right/RConn1 -- PS Divide/LConn2 -- PS Divide2/LConn2
  PS Subtract/LConn1 -- PS Divide1/RConn1
  PS Divide/RConn1 -- PS Subtract/LConn2
  PS Product/LConn1 -- PS-Simulink Converter7/LConn1 -- PS Subtract/RConn1
  stiffness/RConn1 -- PS Product/LConn2
  PS Divide3/RConn1 -- PS Gain1/LConn1
  PS Gain1/RConn1 -- left/RConn1
  right/RConn1 -- PS Divide2/RConn1

== system GVCU_HIL_simscape/vehicle/multibody/Subsystem1 ==
  veh : Inport
  front left : Inport  Port=2
  front right : Inport  Port=3
  rear left : Inport  Port=4
  rear right : Inport  Port=5
  ARB front : Inport  Port=6
  steering front : Inport  Port=7
  steering rear : Inport  Port=8
  ARB rear : Inport  Port=9
  front left contact : Inport  Port=10
  front right contact : Inport  Port=11
  rear left contact : Inport  Port=12
  rear right contact : Inport  Port=13
  Bus Creator{1..4} (4 alike) : BusCreator  Inputs=2
  Bus Creator5 : BusCreator  Inputs=4
  Bus Creator6 : BusCreator  Inputs=4
  Bus Creator8 : BusCreator  Inputs=3
  Out1 : Outport
  wires:
  Bus Creator6/1 -> Bus Creator8/1  "front"
  Bus Creator3/1 -> Bus Creator5/1  "left"
  front left/1 -> Bus Creator1/1
  Bus Creator8/1 -> Out1/1  "vehicle"
  Bus Creator2/1 -> Bus Creator6/2  "right"
  Bus Creator5/1 -> Bus Creator8/2  "rear"
  ARB rear/1 -> Bus Creator5/4  "ARB"
  Bus Creator4/1 -> Bus Creator5/2  "right"
  Bus Creator1/1 -> Bus Creator6/1  "left"
  rear right/1 -> Bus Creator4/1
  front right contact/1 -> Bus Creator2/2
  rear left contact/1 -> Bus Creator3/2
  veh/1 -> Bus Creator8/3
  rear right contact/1 -> Bus Creator4/2
  front left contact/1 -> Bus Creator1/2
  rear left/1 -> Bus Creator3/1
  front right/1 -> Bus Creator2/1
  steering front/1 -> Bus Creator6/4  "steering"
  steering rear/1 -> Bus Creator5/3  "steering"
  ARB front/1 -> Bus Creator6/3  "ARB"

== system GVCU_HIL_simscape/vehicle/multibody/chassis ==
  in : Inport
  " front downforce" : sm_lib/Body Elements/Spherical Solid  SphereRadius=vis.joint.r  SphereRadiusUnits=m  ExportEntireGeometry=off  InertiaType=PointMass  BasedOnType=Density  Density=0  DensityUnits=kg/m^3  Mass=0  MassUnits=kg  CenterOfMass=[0 0 0]  CenterOfMassUnits=m  MomentsOfInertia=[1 1 1]  MomentsOfInertiaUnits=kg*m^2  ProductsOfInertia=[0 0 0]  ProductsOfInertiaUnits=kg*m^2  GraphicType=FromGeometry  MarkerShape=Sphere  MarkerSize=10  GraphicVisPropType=SimpleVisualProperties  GraphicDiffuseColor=vis.joint.color  GraphicOpacity=1  GraphicSpecularColor=[0.5 0.5 0.5 1.0]  GraphicAmbientColor=[0.15 0.15 0.15 1.0]  GraphicEmissiveColor=[0.0 0.0 0.0 1.0]  GraphicShininess=75  DoExposeReferenceFrame=on  SerializedFrames=<Frames/>
  Bus Creator1 : BusCreator  Inputs=4
  Bus Selector : BusSelector  OutputSignals=mFuel
  From3 : From
  Goto3 : Goto
  Rigid Transform1 : sm_lib/Frames and Transforms/Rigid Transform  RotationMethod=None  FollAlignAxisA=+X  BaseAlignAxisA=+Y  FollAlignAxisB=+Y  BaseAlignAxisB=+Z  RotationStandardAxis=+Z  RotationAngle=0  RotationAngleUnits=deg  RotationArbitraryAxis=[0 0 1]  RotationSequenceAxes=FollowerAxes  RotationSequence=XYX  RotationSequenceAngles=[0 0 0]  RotationSequenceAnglesUnits=deg  RotationMatrix=[1 0 0;0 1 0;0 0 1]  Quaternion=[1 0 0 0]  TranslationMethod=Cartesian  TranslationCartesianOffset=front.center.RideF  TranslationCartesianOffsetUnits=m  TranslationStandardAxis=+Z  TranslationStandardOffset=0  TranslationStandardOffsetUnits=m  TranslationROffset=0  TranslationROffsetUnits=m  TranslationThetaOffset=0  TranslationThetaOffsetUnits=deg  TranslationZOffset=0  TranslationZOffsetUnits=m
  Rigid Transform2 : sm_lib/Frames and Transforms/Rigid Transform  RotationMethod=None  FollAlignAxisA=+X  BaseAlignAxisA=+Y  FollAlignAxisB=+Y  BaseAlignAxisB=+Z  RotationStandardAxis=+Z  RotationAngle=0  RotationAngleUnits=deg  RotationArbitraryAxis=[0 0 1]  RotationSequenceAxes=FollowerAxes  RotationSequence=XYX  RotationSequenceAngles=[0 0 0]  RotationSequenceAnglesUnits=deg  RotationMatrix=[1 0 0;0 1 0;0 0 1]  Quaternion=[1 0 0 0]  TranslationMethod=Cartesian  TranslationCartesianOffset=front.center.RideF-veh.CG_sprung  TranslationCartesianOffsetUnits=m  TranslationStandardAxis=+Z  TranslationStandardOffset=0  TranslationStandardOffsetUnits=m  TranslationROffset=0  TranslationROffsetUnits=m  TranslationThetaOffset=0  TranslationThetaOffsetUnits=deg  TranslationZOffset=0  TranslationZOffsetUnits=m
  Rigid Transform3 : sm_lib/Frames and Transforms/Rigid Transform  RotationMethod=None  FollAlignAxisA=+X  BaseAlignAxisA=+Y  FollAlignAxisB=+Y  BaseAlignAxisB=+Z  RotationStandardAxis=+Z  RotationAngle=0  RotationAngleUnits=deg  RotationArbitraryAxis=[0 0 1]  RotationSequenceAxes=FollowerAxes  RotationSequence=XYX  RotationSequenceAngles=[0 0 0]  RotationSequenceAnglesUnits=deg  RotationMatrix=[1 0 0;0 1 0;0 0 1]  Quaternion=[1 0 0 0]  TranslationMethod=Cartesian  TranslationCartesianOffset=rear.center.RideR  TranslationCartesianOffsetUnits=m  TranslationStandardAxis=+Z  TranslationStandardOffset=0  TranslationStandardOffsetUnits=m  TranslationROffset=0  TranslationROffsetUnits=m  TranslationThetaOffset=0  TranslationThetaOffsetUnits=deg  TranslationZOffset=0  TranslationZOffsetUnits=m
  Rigid Transform4 : sm_lib/Frames and Transforms/Rigid Transform  RotationMethod=None  FollAlignAxisA=+X  BaseAlignAxisA=+Y  FollAlignAxisB=+Y  BaseAlignAxisB=+Z  RotationStandardAxis=+Z  RotationAngle=0  RotationAngleUnits=deg  RotationArbitraryAxis=[0 0 1]  RotationSequenceAxes=FollowerAxes  RotationSequence=XYX  RotationSequenceAngles=[0 0 0]  RotationSequenceAnglesUnits=deg  RotationMatrix=[1 0 0;0 1 0;0 0 1]  Quaternion=[1 0 0 0]  TranslationMethod=Cartesian  TranslationCartesianOffset=veh.CG_sprung  TranslationCartesianOffsetUnits=m  TranslationStandardAxis=+Z  TranslationStandardOffset=0  TranslationStandardOffsetUnits=m  TranslationROffset=0  TranslationROffsetUnits=m  TranslationThetaOffset=0  TranslationThetaOffsetUnits=deg  TranslationZOffset=0  TranslationZOffsetUnits=m
  Rigid Transform5 : sm_lib/Frames and Transforms/Rigid Transform  RotationMethod=None  FollAlignAxisA=+X  BaseAlignAxisA=+Y  FollAlignAxisB=+Y  BaseAlignAxisB=+Z  RotationStandardAxis=+Z  RotationAngle=0  RotationAngleUnits=deg  RotationArbitraryAxis=[0 0 1]  RotationSequenceAxes=FollowerAxes  RotationSequence=XYX  RotationSequenceAngles=[0 0 0]  RotationSequenceAnglesUnits=deg  RotationMatrix=[1 0 0;0 1 0;0 0 1]  Quaternion=[1 0 0 0]  TranslationMethod=Cartesian  TranslationCartesianOffset=rear.center.RideR-veh.CG_sprung  TranslationCartesianOffsetUnits=m  TranslationStandardAxis=+Z  TranslationStandardOffset=0  TranslationStandardOffsetUnits=m  TranslationROffset=0  TranslationROffsetUnits=m  TranslationThetaOffset=0  TranslationThetaOffsetUnits=deg  TranslationZOffset=0  TranslationZOffsetUnits=m
  Subsystem : Subsystem
      settings: PortSchema="{\"entries\":[{\"content\":{\"sides\":[{\"content\":{\"connectorIds\":[\"LConn1\",\"LConn2\",\"LConn3\"]},\"type\":\"ConnectorPlacement.EquallySpacedRectSide\",\"uuid\":\"dbef32a1-2cd0-444b-91fe-3fbfb2345183\"},{\"content\":{\"side\":\"RIGHT\"},\"type\":\"ConnectorPlacement.EquallySpacedRectSide\",\"uuid\":\"aa4879d0-5b71-4cf5-8af3-1de8821aa310\"},{\"content\":{\"side\":\"TOP\"},\"type\":\"ConnectorPlacement.EquallySpacedRectSide\",\"uuid\":\"39100a88-bef5-4db8-8f68-733ba7e4106b\"},{\"content\":{\"connectorIds\":[\"Out1\",\"Out2\"],\"side\":\"BOTTOM\"},\"type\":\"ConnectorPlacement.EquallySpacedRectSide\",\"uuid\":\"95e7d766-de8e-4ee9-8dac-970b0bf9ede2\"}]},\"type\":\"ConnectorPlacement.EquallySpacedConnector\",\"uuid\":\"ec50e4e1-dcdd-4c06-91fd-7d8bc33d68d0\"}],\"packageUris\":[\"http://schema.mathworks.com/mf0/Connector/R2020b\"],\"version\":\"1.0\"}"
  Subsystem1 : Subsystem
  Terminator : Terminator
  body : Subsystem  VariantControl=config.vehicle.model == 2
      settings: PortSchema="{\"entries\":[{\"content\":{\"sides\":[{\"content\":{},\"type\":\"ConnectorPlacement.EquallySpacedRectSide\",\"uuid\":\"e6e4ed55-fd58-4138-9282-a613b9bb7ca2\"},{\"content\":{\"side\":\"RIGHT\"},\"type\":\"ConnectorPlacement.EquallySpacedRectSide\",\"uuid\":\"dae26dfd-24a9-4dae-ba70-c3841055d2ae\"},{\"content\":{\"side\":\"TOP\"},\"type\":\"ConnectorPlacement.EquallySpacedRectSide\",\"uuid\":\"d5e7ccf3-a2f4-47e2-9100-528b9fb6f658\"},{\"content\":{\"connectorIds\":[\"RConn1\"],\"side\":\"BOTTOM\"},\"type\":\"ConnectorPlacement.EquallySpacedRectSide\",\"uuid\":\"8b3655fe-699d-4c60-be5e-022fe2c82b2b\"}]},\"type\":\"ConnectorPlacement.EquallySpacedConnector\",\"uuid\":\"23e0293c-f657-4357-ae54-7e75cba69bdb\"}],\"packageUris\":[\"http://schema.mathworks.com/mf0/Connector/R2020b\"],\"version\":\"1.0\"}"
  dynamic cameras : Subsystem
      settings: PortSchema="{\"entries\":[{\"content\":{\"sides\":[{\"content\":{},\"type\":\"ConnectorPlacement.EquallySpacedRectSide\",\"uuid\":\"929363c8-be46-44fb-b764-f7d2bc908c8c\"},{\"content\":{\"side\":\"RIGHT\"},\"type\":\"ConnectorPlacement.EquallySpacedRectSide\",\"uuid\":\"9512f6c6-fafb-4645-a591-b6909a7b4996\"},{\"content\":{\"side\":\"TOP\"},\"type\":\"ConnectorPlacement.EquallySpacedRectSide\",\"uuid\":\"5047d8a4-a182-4e52-847f-a162a06ecd08\"},{\"content\":{\"connectorIds\":[\"RConn1\"],\"side\":\"BOTTOM\"},\"type\":\"ConnectorPlacement.EquallySpacedRectSide\",\"uuid\":\"918eb3d5-7efc-4d68-8af9-2bb4d67a38a7\"}]},\"type\":\"ConnectorPlacement.EquallySpacedConnector\",\"uuid\":\"94548d94-0a61-4586-8067-75ed5bf59e67\"}],\"packageUris\":[\"http://schema.mathworks.com/mf0/Connector/R2020b\"],\"version\":\"1.0\"}"
  local coordinates : Subsystem
  rear downforce : sm_lib/Body Elements/Spherical Solid  SphereRadius=vis.joint.r  SphereRadiusUnits=m  ExportEntireGeometry=off  InertiaType=PointMass  BasedOnType=Density  Density=0  DensityUnits=kg/m^3  Mass=0  MassUnits=kg  CenterOfMass=[0 0 0]  CenterOfMassUnits=m  MomentsOfInertia=[1 1 1]  MomentsOfInertiaUnits=kg*m^2  ProductsOfInertia=[0 0 0]  ProductsOfInertiaUnits=kg*m^2  GraphicType=FromGeometry  MarkerShape=Sphere  MarkerSize=10  GraphicVisPropType=SimpleVisualProperties  GraphicDiffuseColor=vis.joint.color  GraphicOpacity=1  GraphicSpecularColor=[0.5 0.5 0.5 1.0]  GraphicAmbientColor=[0.15 0.15 0.15 1.0]  GraphicEmissiveColor=[0.0 0.0 0.0 1.0]  GraphicShininess=75  DoExposeReferenceFrame=on  SerializedFrames=<Frames/>
  vehicle mass and inertia : sm_lib/Body Elements/Spherical Solid  SphereRadius=0.02  SphereRadiusUnits=m  ExportEntireGeometry=off  InertiaType=Custom  BasedOnType=Density  Density=1000  DensityUnits=kg/m^3  Mass=veh.m  MassUnits=kg  CenterOfMass=[0 0 0]  CenterOfMassUnits=m  MomentsOfInertia=veh.I  MomentsOfInertiaUnits=kg*m^2  ProductsOfInertia=[0 0 0]  ProductsOfInertiaUnits=kg*m^2  GraphicType=FromGeometry  MarkerShape=Sphere  MarkerSize=10  GraphicVisPropType=SimpleVisualProperties  GraphicDiffuseColor=[0.5 0.5 0.5]  GraphicOpacity=1  GraphicSpecularColor=[0.5 0.5 0.5 1.0]  GraphicAmbientColor=[0.15 0.15 0.15 1.0]  GraphicEmissiveColor=[0.0 0.0 0.0 1.0]  GraphicShininess=75  DoExposeReferenceFrame=on  SerializedFrames=<Frames/>
  ref : PMIOPort  Side=Left
  front : PMIOPort  Port=2  Side=Left
  rear : PMIOPort  Port=3  Side=Right
  meas : Outport
  wires:
  Subsystem1/1(meas) -> Goto3/1
  [B] -> Bus Creator1/2
  Bus Creator1/1 -> meas/1  "veh"
  From3/1 -> Bus Creator1/1
  local coordinates/1(meas) -> [B]
  Subsystem/2(meas1) -> [D]
  Subsystem/1(meas) -> [C]
  [C] -> Bus Creator1/3
  [D] -> Bus Creator1/4
  in/1 -> Bus Selector/1
  Bus Selector/1 -> Terminator/1  "<mFuel>"
  connections:
  rear/RConn1 -- Rigid Transform3/LConn1
  front/RConn1 -- Rigid Transform1/LConn1
  Rigid Transform2/RConn1 -- Subsystem/LConn1 -- " front downforce"/RConn1 -- Rigid Transform1/RConn1
  Rigid Transform5/RConn1 -- Subsystem/LConn3 -- rear downforce/RConn1 -- Rigid Transform3/RConn1
  Rigid Transform4/LConn1 -- ref/RConn1
  Subsystem/LConn2 -- Rigid Transform2/LConn1 -- Rigid Transform5/LConn1 -- vehicle mass and inertia/RConn1 -- body/RConn1 -- dynamic cameras/RConn1 -- Subsystem1/RConn1 -- local coordinates/LConn1
  Subsystem1/LConn1 -- Rigid Transform4/RConn1
